simulink model "Arm_2DOF"  (R2021a)
settings: Solver=VariableStepAuto  StartTime=0.0  StopTime=10.0  RelTol=1e-3
Description:
  | Model for a 2DOF Arm Robot
settings Model: Creator=Zicx  LastModifiedBy=Zicx
settings DataIOCC: SaveOutput=off  SaveTime=off

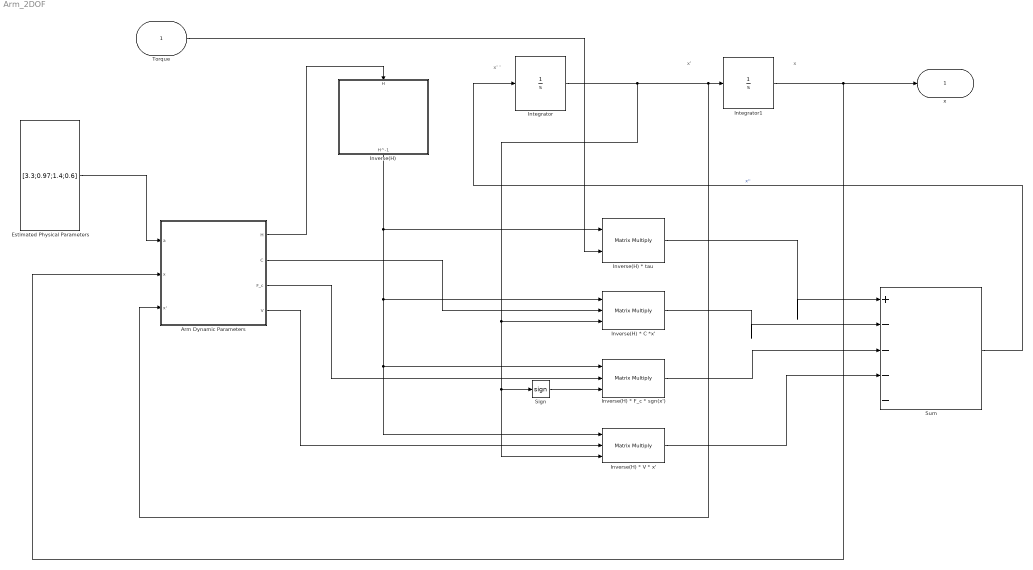
== system Arm_2DOF ==
  note: x
  note: x'
  note: x' '
  Torque : Inport  OutDataTypeStr=double  PortDimensions=[2 1]
  Arm Dynamic Parameters : Subsystem
  Estimated Physical Parameters : Constant  Value=[3.3;0.97;1.4;0.6]
  Integrator : Integrator  InitialCondition=[0;0]
  Integrator1 : Integrator  InitialCondition=[0.3;0.5]  ContinuousStateAttributes='position'
  Inverse(H) : Subsystem
  Inverse(H) * C *x' : Product  Inputs=3  Multiplication=Matrix(*)
  Inverse(H) * F_c * sgn(x') : Product  Inputs=3  Multiplication=Matrix(*)
  Inverse(H) * V * x' : Product  Inputs=3  Multiplication=Matrix(*)
  Inverse(H) * tau : Product  Multiplication=Matrix(*)
  Sign : Signum  ZeroCross=off
  Sum : Sum  Inputs=|+----
  x : Outport  SignalName=x  OutDataTypeStr=double  PortDimensions=[2 1]  SampleTime=0
  wires:
  Inverse(H) * V * x'/1 -> Sum/4
  Inverse(H) * F_c * sgn(x')/1 -> Sum/3
  Inverse(H) * C *x'/1 -> Sum/2
  Torque/1 -> Inverse(H) * tau/2
  Inverse(H) * tau/1 -> Sum/1
  Estimated Physical Parameters/1 -> Arm Dynamic Parameters/1(a)
  Inverse(H)/1(H^-1) -> Inverse(H) * tau/1, Inverse(H) * C *x'/1, Inverse(H) * F_c * sgn(x')/1, Inverse(H) * V * x'/1
  Sum/1 -> Integrator/1  "x''"
  Integrator1/1 -> x/1, Arm Dynamic Parameters/2(x)
  Integrator/1 -> Inverse(H) * C *x'/3, Inverse(H) * V * x'/3, Sign/1, Arm Dynamic Parameters/3(x'), Integrator1/1
  Arm Dynamic Parameters/1(H) -> Inverse(H)/1(H)
  Arm Dynamic Parameters/2(C) -> Inverse(H) * C *x'/2
  Arm Dynamic Parameters/3(F_c) -> Inverse(H) * F_c * sgn(x')/2
  Arm Dynamic Parameters/4(V) -> Inverse(H) * V * x'/2
  Sign/1 -> Inverse(H) * F_c * sgn(x')/3

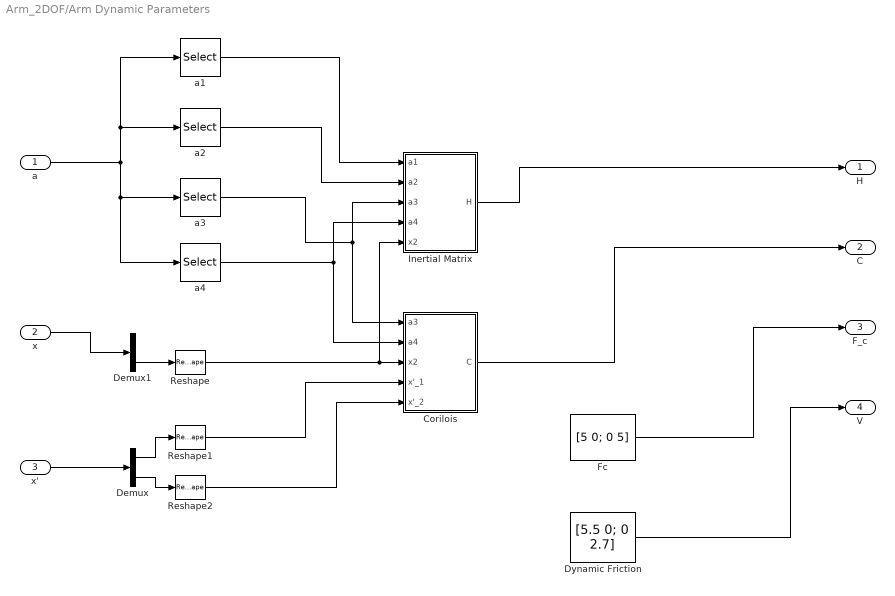
== system Arm_2DOF/Arm Dynamic Parameters ==
  a : Inport
  x : Inport  Port=2  PortDimensions=[2 1]
  x' : Inport  Port=3  PortDimensions=[2 1]
  Corilois : Subsystem
  Demux : Demux  Outputs=2
  Demux1 : Demux  Outputs=2
  Dynamic Friction : Constant  Value=[5.5 0; 0 2.7]
  Fc : Constant  Value=[5 0; 0 5]
  Inertial Matrix : Subsystem
  Reshape : Reshape  OutputDimensionality=Customize  OutputDimensions=1
  Reshape1 : Reshape  OutputDimensionality=Customize  OutputDimensions=1
  Reshape2 : Reshape  OutputDimensionality=Customize  OutputDimensions=1
  a1 : Selector  InputPortWidth=4  IndexOptions=Index vector (dialog)  Indices=[1]  OutputSizes=1
  a2 : Selector  InputPortWidth=4  IndexOptions=Index vector (dialog)  Indices=[2]  OutputSizes=1
  a3 : Selector  InputPortWidth=4  IndexOptions=Index vector (dialog)  Indices=[3]  OutputSizes=1
  a4 : Selector  InputPortWidth=4  IndexOptions=Index vector (dialog)  Indices=[4]  OutputSizes=1
  H : Outport
  C : Outport  Port=2
  F_c : Outport  Port=3
  V : Outport  Port=4
  wires:
  a1/1 -> Inertial Matrix/1(a1)
  a/1 -> a1/1, a2/1, a4/1, a3/1
  a3/1 -> Corilois/1(a3), Inertial Matrix/3(a3)
  a4/1 -> Inertial Matrix/4(a4), Corilois/2(a4)
  a2/1 -> Inertial Matrix/2(a2)
  Inertial Matrix/1(H) -> H/1
  Corilois/1(C) -> C/1
  x/1 -> Demux1/1
  Fc/1 -> F_c/1
  Dynamic Friction/1 -> V/1
  x'/1 -> Demux/1
  Demux1/2 -> Reshape/1
  Reshape/1 -> Inertial Matrix/5(x2), Corilois/3(x2)
  Demux/1 -> Reshape1/1
  Demux/2 -> Reshape2/1
  Reshape1/1 -> Corilois/4(x'_1)
  Reshape2/1 -> Corilois/5(x'_2)

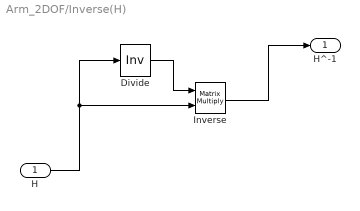
== system Arm_2DOF/Inverse(H) ==
  H : Inport  PortDimensions=[2 2]
  Divide : Product  Inputs=/  Multiplication=Matrix(*)
  Inverse : Product  Multiplication=Matrix(*)
  H^-1 : Outport
  wires:
  Divide/1 -> Inverse/1
  Inverse/1 -> H^-1/1
  H/1 -> Inverse/2, Divide/1

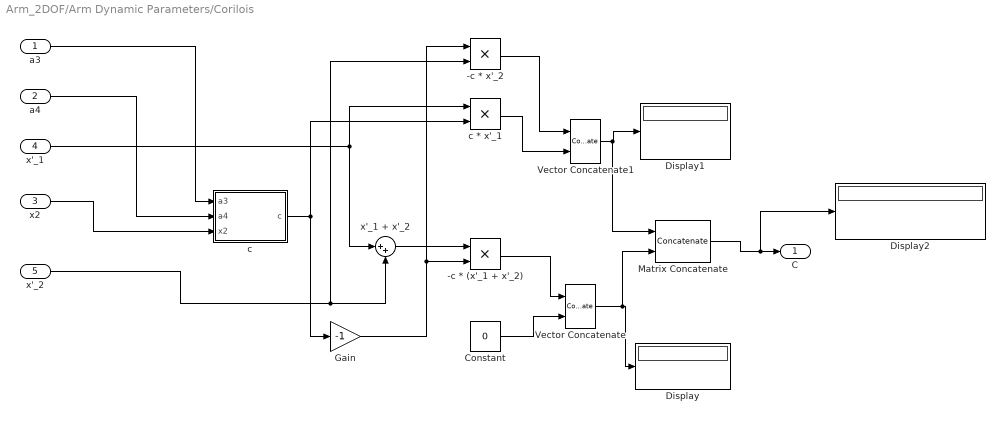
== system Arm_2DOF/Arm Dynamic Parameters/Corilois ==
  a3 : Inport
  a4 : Inport  Port=2
  x2 : Inport  Port=3
  x'_1 : Inport  Port=4
  x'_2 : Inport  Port=5
  -c * (x'_1 + x'_2) : Product
  -c * x'_2 : Product
  Constant : Constant  Value=0
  Display : Display
  Display1 : Display
  Display2 : Display
  Gain : Gain  Gain=-1
  Matrix Concatenate : Concatenate  Mode=Multidimensional array  ConcatenateDimension=2
  Vector Concatenate : Concatenate
  Vector Concatenate1 : Concatenate
  c : MATLAB Function  TreatAsAtomicUnit=on
  c * x'_1 : Product
  x'_1 + x'_2 : Sum  Inputs=|++
  C : Outport
  wires:
  Matrix Concatenate/1 -> Display2/1, C/1
  a4/1 -> c/2(a4)
  a3/1 -> c/1(a3)
  Vector Concatenate1/1 -> Matrix Concatenate/1, Display1/1
  x'_1/1 -> x'_1 + x'_2/1, c * x'_1/1
  x2/1 -> c/3(x2)
  c/1(c) -> c * x'_1/2, Gain/1
  x'_2/1 -> x'_1 + x'_2/2, -c * x'_2/2
  x'_1 + x'_2/1 -> -c * (x'_1 + x'_2)/1
  Vector Concatenate/1 -> Matrix Concatenate/2, Display/1
  Gain/1 -> -c * x'_2/1, -c * (x'_1 + x'_2)/2
  -c * x'_2/1 -> Vector Concatenate1/1
  c * x'_1/1 -> Vector Concatenate1/2
  -c * (x'_1 + x'_2)/1 -> Vector Concatenate/1
  Constant/1 -> Vector Concatenate/2

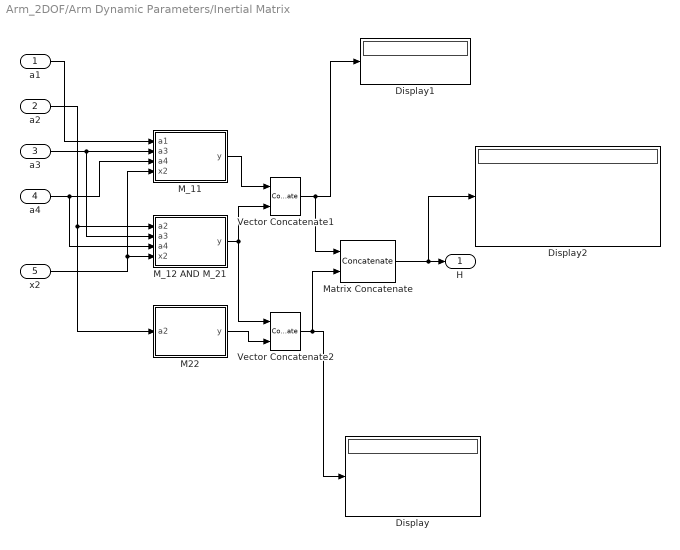
== system Arm_2DOF/Arm Dynamic Parameters/Inertial Matrix ==
  a1 : Inport
  a2 : Inport  Port=2
  a3 : Inport  Port=3
  a4 : Inport  Port=4
  x2 : Inport  Port=5
  Display : Display
  Display1 : Display
  Display2 : Display
  M22 : MATLAB Function  TreatAsAtomicUnit=on
  M_11 : MATLAB Function  TreatAsAtomicUnit=on
  M_12 AND M_21 : MATLAB Function  TreatAsAtomicUnit=on
  Matrix Concatenate : Concatenate  Mode=Multidimensional array  ConcatenateDimension=2
  Vector Concatenate1 : Concatenate
  Vector Concatenate2 : Concatenate
  H : Outport
  wires:
  Matrix Concatenate/1 -> Display2/1, H/1
  a1/1 -> M_11/1(a1)
  a3/1 -> M_11/2(a3), M_12 AND M_21/2(a3)
  a4/1 -> M_11/3(a4), M_12 AND M_21/3(a4)
  a2/1 -> M22/1(a2), M_12 AND M_21/1(a2)
  Vector Concatenate2/1 -> Display/1, Matrix Concatenate/2
  M22/1(y) -> Vector Concatenate2/2
  Vector Concatenate1/1 -> Display1/1, Matrix Concatenate/1
  M_12 AND M_21/1(y) -> Vector Concatenate2/1, Vector Concatenate1/2
  x2/1 -> M_12 AND M_21/4(x2), M_11/4(x2)
  M_11/1(y) -> Vector Concatenate1/1

== matlab function Arm_2DOF/Arm Dynamic Parameters/Corilois/c ==
  data: a3 input; c output; a4 input; x2 input
function c = fcn(a3, a4, x2)

c = a3 * sin(x2) - a4 * cos(x2);

== matlab function Arm_2DOF/Arm Dynamic Parameters/Inertial Matrix/M22 ==
  data: a2 input; y output
function y = fcn(a2)

y = a2;

== matlab function Arm_2DOF/Arm Dynamic Parameters/Inertial Matrix/M_11 ==
  data: a1 input; a3 input; a4 input; y output; x2 input
function y = fcn(a1, a3, a4, x2)
%#codegen

y = a1 + 2*a3 * cos(x2)- 2 * a4 * sin(x2);

== matlab function Arm_2DOF/Arm Dynamic Parameters/Inertial Matrix/M_12 AND M_21 ==
  data: a2 input; y output; a3 input; a4 input; x2 input
function y = fcn(a2, a3, a4, x2)

y = a2 + a3 * cos(x2) + a4 * sin(x2);
